simulink model "cstr_control_loops"  (R2019a)
settings: Solver=ode15s  StartTime=0.0  StopTime=450  RelTol=1e-3
values from neighbouring files (symbols this model uses):
  cstr_const =     [matlab.mat]    (also in prepare_sim.m = struct(); withnmpc.mat)
settings Model: Creator=User  LastModifiedBy=User
settings DebuggingCC: PregeneratedLibrarySubsystemCodeDiagnostic=none  ArithmeticOperatorsInVariantConditions=warning
settings CodeAppCC: StateflowObjectComments=on

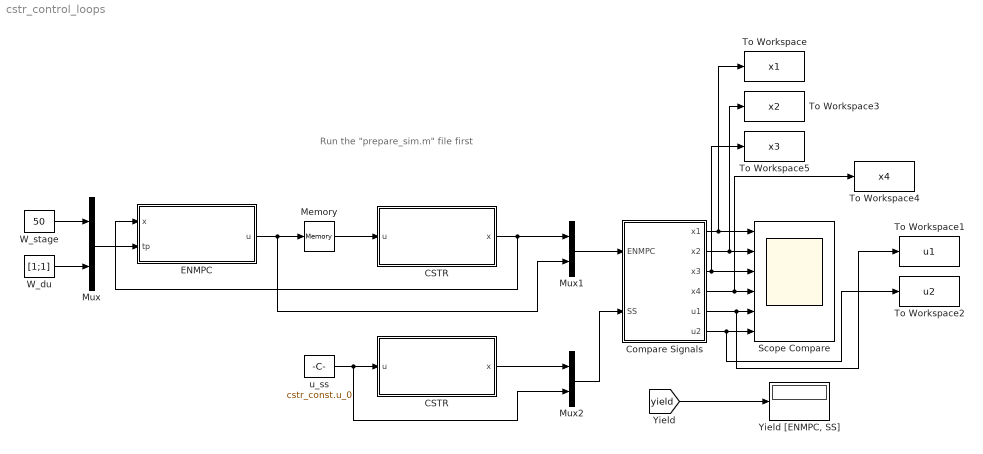
== system cstr_control_loops ==
  note: Run the "prepare_sim.m" file first
  " CSTR " : Subsystem
  " Yield [ENMPC, SS]" : Display
  CSTR : Subsystem
  Compare Signals : Subsystem
  ENMPC : Subsystem
  Memory : Memory  InitialCondition=cstr_const.u_0
  Mux : Mux  Inputs=2
  Mux1 : Mux  Inputs=2
  Mux2 : Mux  Inputs=2
  Scope Compare : Scope  NumInputPorts=6
  To Workspace : ToWorkspace  VariableName=x1  SaveFormat=Structure With Time  SampleTime=-1
  To Workspace1 : ToWorkspace  VariableName=u1  SaveFormat=Structure With Time  SampleTime=-1
  To Workspace2 : ToWorkspace  VariableName=u2  SaveFormat=Structure With Time  SampleTime=-1
  To Workspace3 : ToWorkspace  VariableName=x2  SaveFormat=Structure With Time  SampleTime=-1
  To Workspace4 : ToWorkspace  VariableName=x4  SaveFormat=Structure With Time  SampleTime=-1
  To Workspace5 : ToWorkspace  VariableName=x3  SaveFormat=Structure With Time  SampleTime=-1
  W_du : Constant  Value=[1;1]
  W_stage : Constant  Value=50
  u_ss : Constant  Value=cstr_const.u_0
  wires:
  ENMPC/1(u) -> Mux1/2, Memory/1
  CSTR/1(x) -> ENMPC/1(x), Mux1/1
  W_stage/1 -> Mux/1
  Mux/1 -> ENMPC/2(tp)
  [yield] -> " Yield [ENMPC, SS]"/1
  Memory/1 -> CSTR/1(u)
  Mux1/1 -> Compare Signals/1(ENMPC)
  " CSTR "/1(x) -> Mux2/1
  u_ss/1 -> " CSTR "/1(u), Mux2/2
  W_du/1 -> Mux/2
  Mux2/1 -> Compare Signals/2(SS)
  Compare Signals/1(x1) -> To Workspace/1, Scope Compare/1
  Compare Signals/2(x2) -> To Workspace3/1, Scope Compare/2
  Compare Signals/5(u1) -> To Workspace1/1, Scope Compare/5
  Compare Signals/6(u2) -> To Workspace2/1, Scope Compare/6
  Compare Signals/3(x3) -> Scope Compare/3, To Workspace5/1
  Compare Signals/4(x4) -> Scope Compare/4, To Workspace4/1

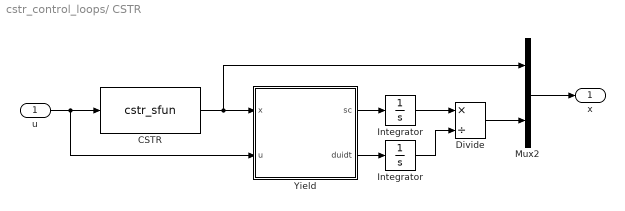
== system cstr_control_loops/ CSTR  ==
  u : Inport
  " Integrator " : Integrator
  CSTR : S-Function  FunctionName=cstr_sfun  SFunctionDeploymentMode=off  EnableBusSupport=off
  Divide : Product  Inputs=*/
  Integrator : Integrator
  Mux2 : Mux  Inputs=2
  Yield : MATLAB Function  TreatAsAtomicUnit=on
  x : Outport
  wires:
  u/1 -> Yield/2(u), CSTR/1
  CSTR/1 -> Mux2/1, Yield/1(x)
  Mux2/1 -> x/1
  Yield/1(sc) -> Integrator/1
  Yield/2(duidt) -> " Integrator "/1
  Integrator/1 -> Divide/1
  " Integrator "/1 -> Divide/2
  Divide/1 -> Mux2/2

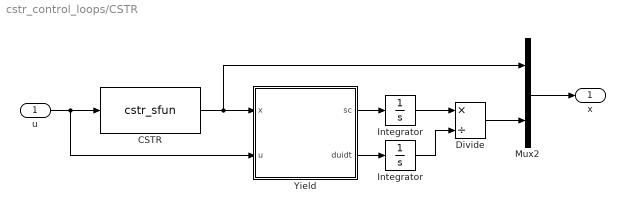
== system cstr_control_loops/CSTR ==
  u : Inport
  " Integrator " : Integrator
  CSTR : S-Function  FunctionName=cstr_sfun  SFunctionDeploymentMode=off  EnableBusSupport=off
  Divide : Product  Inputs=*/
  Integrator : Integrator
  Mux2 : Mux  Inputs=2
  Yield : MATLAB Function  TreatAsAtomicUnit=on
  x : Outport
  wires:
  u/1 -> Yield/2(u), CSTR/1
  CSTR/1 -> Mux2/1, Yield/1(x)
  Mux2/1 -> x/1
  Yield/1(sc) -> Integrator/1
  Yield/2(duidt) -> " Integrator "/1
  Integrator/1 -> Divide/1
  " Integrator "/1 -> Divide/2
  Divide/1 -> Mux2/2

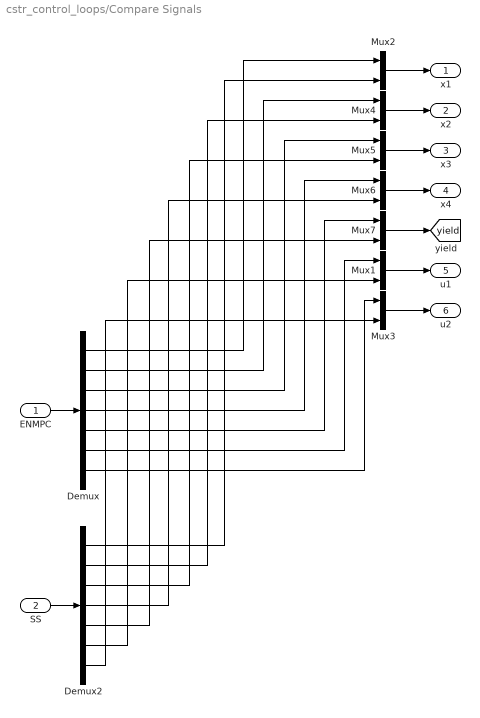
== system cstr_control_loops/Compare Signals ==
  ENMPC : Inport
  SS : Inport  Port=2
  Demux : Demux  Outputs=7
  Demux2 : Demux  Outputs=7
  Mux{1..7} (7 alike) : Mux  Inputs=2
  x1 : Outport
  x2 : Outport  Port=2
  x3 : Outport  Port=3
  x4 : Outport  Port=4
  u1 : Outport  Port=5
  u2 : Outport  Port=6
  tag scope: yield=global
  wires:
  ENMPC/1 -> Demux/1
  Demux/2 -> Mux4/1
  Demux/1 -> Mux2/1
  SS/1 -> Demux2/1
  Demux2/1 -> Mux2/2
  Demux2/2 -> Mux4/2
  Demux/3 -> Mux5/1
  Demux2/3 -> Mux5/2
  Demux/4 -> Mux6/1
  Demux2/4 -> Mux6/2
  Demux/5 -> Mux7/1
  Demux2/5 -> Mux7/2
  Demux/6 -> Mux1/1
  Demux2/6 -> Mux1/2
  Demux/7 -> Mux3/1
  Demux2/7 -> Mux3/2
  Mux3/1 -> u2/1
  Mux1/1 -> u1/1
  Mux6/1 -> x4/1
  Mux5/1 -> x3/1
  Mux4/1 -> x2/1
  Mux2/1 -> x1/1
  Mux7/1 -> [yield]

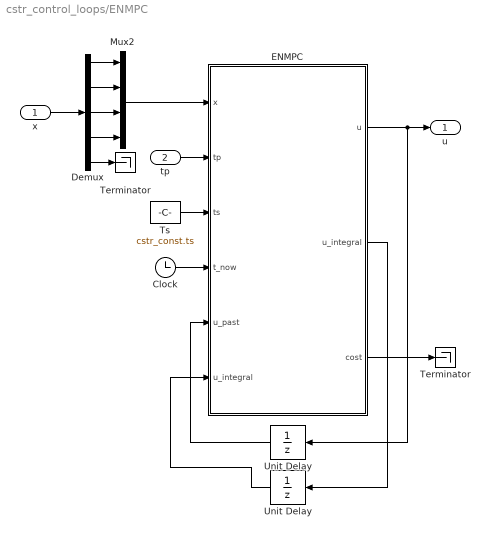
== system cstr_control_loops/ENMPC ==
  x : Inport
  tp : Inport  Port=2
  " Unit Delay " : UnitDelay  SampleTime=cstr_const.ts  HasFrameUpgradeWarning=on
  Clock : Clock
  Demux : Demux  Outputs=5
  "ENMPC " : MATLAB Function  TreatAsAtomicUnit=on  SystemSampleTime=cstr_const.ts
  Mux2 : Mux
  Terminator : Terminator
  "Terminator " : Terminator
  Ts : Constant  Value=cstr_const.ts
  Unit Delay : UnitDelay  InitialCondition=cstr_const.u_0  SampleTime=cstr_const.ts  HasFrameUpgradeWarning=on
  u : Outport
  wires:
  "ENMPC "/1(u) -> Unit Delay/1, u/1
  Unit Delay/1 -> "ENMPC "/5(u_past)
  x/1 -> Demux/1
  tp/1 -> "ENMPC "/2(tp)
  Ts/1 -> "ENMPC "/3(ts)
  "ENMPC "/3(cost) -> "Terminator "/1
  Mux2/1 -> "ENMPC "/1(x)
  Demux/5 -> Terminator/1
  Clock/1 -> "ENMPC "/4(t_now)
  " Unit Delay "/1 -> "ENMPC "/6("u_integral ")
  "ENMPC "/2(u_integral) -> " Unit Delay "/1
  Demux/4 -> Mux2/4
  Demux/3 -> Mux2/3
  Demux/2 -> Mux2/2
  Demux/1 -> Mux2/1

== matlab function cstr_control_loops/ENMPC/ENMPC  ==
  data: u output size=[2,1]; u_integral output; cost output size=[1,1]; x input; tp input; ts input; t_now input; u_past input; u_integral input
function [u, u_integral, cost] = enmpc(x,tp,ts,t_now,u_past,u_integral)
    u = u_past; cost = 0;
    coder.extrinsic('get_control_input');
    [u, u_integral, cost] = get_control_input(x, u_past, tp, u_integral, t_now, 1, ts);
end

== matlab function cstr_control_loops/ CSTR /Yield ==
  data: x input; u input; sc output; duidt output
function [sc, duidt] = cost(x,u)
    sc = 0; duidt = 1e-4;
    coder.extrinsic('ode_set');
    [~,sc,duidt] = ode_set(x,u);
end

== matlab function cstr_control_loops/CSTR/Yield ==
  data: x input; u input; sc output; duidt output
function [sc, duidt] = cost(x,u)
    sc = 0; duidt = 1e-4;
    coder.extrinsic('ode_set');
    [~,sc,duidt] = ode_set(x,u);
end
